simulink model "DUC_filters"  (R2014b)
settings: Solver=FixedStepDiscrete  SolverMode=SingleTasking  StartTime=0.0  StopTime=4096/fs  RelTol=1e-3
PreLoadFcn:
  | %%%%%%%%%%%%%%%%%%%%%%%%%%%%%%%%%%%%%%%%%%%%%%%%%%%%%%%%%%%%%%%%%%%%%%%%%%%
  | % check to see if Simulink library folder is missing from the MATLAB path %
  | %%%%%%%%%%%%%%%%%%%%%%%%%%%%%%%%%%%%%%%%%%%%%%%%%%%%%%%%%%%%%%%%%%%%%%%%%%%
  | if isempty(strfind(path, 'rtlsdr_book_library'))
  | 
  |     % create error window
  |     fig_error = figure(...
  |         'Name', 'Error: RTL-SDR Book Library',...
  |         'Toolbar','none',...
  |         'MenuBar','none',...
  |         'NumberTitle','off',...
  |         'Resize','off',...
  |         'WindowStyle','modal');
  |     fig_error.Position(3) = 600;
  |     fig_error.Position(4) = 150;
  |     fig_axes = axes(...
  |         'Parent',fig_error,...
  |         'Position',[0,0,1,1],...
  |         'visible','off');
  |     % error message
  |     t_title = text(.05,.8,...
  |         'MISSING DIRECTORIES',...
  |         'FontSize',11.5);
  |     t_body = text(.075,.6,...
  |         [{'Simulink cannot find the  \it{<root>}\rm / \it{rtlsdr\_book\_library}\rm  folder in the \it{MATLAB Path}\rm.'},...
  |         {'Please set the MATLAB path following the instructions given in Exercise 2.4.'}],...
  |         'FontSize',10.5);
  |     % buttons
  |     btn_path = uicontrol(...
  |         'Parent',fig_error,...
  |         'String','Set Path Now',...
  |         'FontSize',10,...
  |         'Callback', 'pathtool; close(fig_error);',...
  |         'Position', [fig_error.Position(3)/2-210, 30, 200, 30]);
  |     btn_abort = uicontrol(...
  |         'Parent',fig_error,...
  |         'String','No thanks',...
  |         'FontSize',10,...
  |         'Callback', 'close(fig_error); abort=1;',...
  |         'Position', [fig_error.Position(3)/2+10, 30, 200, 30]);
  | 
  |     % pause to allow user to interact with error box
  |     uiwait(fig_error);
  | 
  |     % abort simulation
  |     try
  |         if abort==1
  |             set_param(gcs, 'SimulationCommand', 'stop');
  |         end
  |     end
  | 
  |     % if user has set path, allow diagram to be updated
  |     if ~exist('abort','var')
  |         % create error window
  |         fig_update = figure(...
  |             'Name', 'Update Diagram',...
  |             'Toolbar','none',...
  |             'MenuBar','none',...
  |             'NumberTitle','off',...
  |             'Resize','off');
  |         fig_update.Position(3) = 400;
  |         fig_update.Position(4) = 120;
  |         fig_axes = axes(...
  |             'Parent',fig_update,...
  |             'Position',[0,0,1,1],...
  |             'visible','off');
  |         % instruction message
  |         t_body = text(.075,.7,...
  |             'Once you have set the path, update the block diagram',...
  |             'FontSize',10.5);
  |         % button
  |         btn_update = uicontrol(...
  |             'Parent',fig_update,...
  |             'String','Update Block Diagram',...
  |             'FontSize',10,...
  |             'Callback', 'set_param(gcs,''SimulationCommand'',''update''); close(gcf)',...
  |             'Position', [fig_update.Position(3)/2-100, 30, 200, 30]);
  |     end
  | 
  |     % clear error components
  |     clear('fig_error','fig_update','fig_axes','t_title','t_body','btn_path','btn_abort','btn_update','abort');
  | 
  | end
  | %%%%%%%%%%%%%%%%%%%%%%%%%%%%%%%%%%%%%%%%%%%%%%%%%%%%%%%%%%%%%%%%%%%%%%%%%%%
  | 
  | DUC1_setup
  | 
  | % annotations for the pink and purple blocks
  | % going from right to left...
  | 
  | MHz = 100;
  | fs = MHz * 1e6;
  | 
  | fs_CIC_in = fs/CIC_R;
  | MHz_CIC_in = MHz/CIC_R;
  | 
  | fs_CFIR_in = fs/(CIC_R*CFIR_L_factor);
  | MHz_CFIR_in = MHz/(CIC_R*CFIR_L_factor);
  | 
  | fs_RRC_in = fs/(CIC_R*CFIR_L_factor*RRC_L_factor);
  | MHz_RRC_in = MHz/(CIC_R*CFIR_L_factor*RRC_L_factor);
StartFcn:
  | close all;
undefined symbols (not defined in the file): CFIR_L_factor, CIC_R, K_cic, RRC_L_factor, startfcn_spectrum_analyzer, startfcn_time_scope
libraries: dspmlti4 x6, rtlsdr_book_library x1, commdigbbndpm3 x1, commrandsrc2 x1, dspsigops x1
CloseFcn:
  | closefcn_model;
Description:
  | Software, Simulation Examples and Design Exercises Licence Agreement
  | 
  | This license agreement refers to the simulation examples, design exercises and files,
  | and associated software MATLAB and Simulink resources that accompany the book:
  | 
  |      Title: Software Defined Radio using MATLAB & Simulink and the RTL-SDR
  |      Published by Strathclyde Academic Media, 2015
  |      Authored by Robert W. Stewart, Kenneth W. Barlee, Dale S.W. Atkinson,
  |      and Louise H. Crockett
  | 
  | and made available as a download from, www.desktopSDR.com or variously acquired
  | by other means such as via USB storage, cloud storage, disk or any other electronic
  | or optical or magnetic storage mechanism. These files and associated software may
  | be used subject to the terms of agreement of the conditions below:
  | 
  |     Copyright © 2015 Robert W. Stewart, Kenneth W. Barlee, Dale S.W. Atkinson,
  |     and Louise H. Crockett
  |     All rights reserved.
  | 
  | Redistribution and use in source and binary forms, with or without modification, are
  | permitted provided that the following conditions are met:
  | 
  |    1.  Redistributions of source code must retain the above copyright notice, this list of
  |         conditions and the following disclaimer.
  | 
  |    2.  Redistributions in binary form must reproduce the above copyright notice, this
  |         list of conditions and the following disclaimer in the documentation and/or other
  |         materials provided with the distribution.
  | 
  |    3.  Neither the name of the copyright holder nor the names of its contributors may
  |         be used to endorse or promote products derived from this software without
  |         specific prior written permission.
  | 
  |    4.  In all cases, the software is, and all modifications and derivatives of the
  |         software shall be, licensed to you solely for use in conjunction with The
  |         MathWorks, Inc. products and service offerings.
  | 
  | THIS SOFTWARE IS PROVIDED BY THE COPYRIGHT HOLDERS AND CONTRIBUTORS
  | "AS IS" AND ANY EXPRESS OR IMPLIED WARRANTIES, INCLUDING, BUT NOT LIMITED
  | TO, THE IMPLIED WARRANTIES OF MERCHANTABILITY AND FITNESS FOR A
  | PARTICULAR PURPOSE ARE DISCLAIMED. IN NO EVENT SHALL THE COPYRIGHT
  | HOLDER OR CONTRIBUTORS BE LIABLE FOR ANY DIRECT, INDIRECT, INCIDENTAL,
  | SPECIAL, EXEMPLARY, OR CONSEQUENTIAL DAMAGES (INCLUDING, BUT NOT
  | LIMITED TO, PROCUREMENT OF SUBSTITUTE GOODS OR SERVICES; LOSS OF USE,
  | DATA, OR PROFITS; OR BUSINESS INTERRUPTION) HOWEVER CAUSED AND ON ANY
  | THEORY OF LIABILITY, WHETHER IN CONTRACT, STRICT LIABILITY, OR TORT
  | (INCLUDING NEGLIGENCE OR OTHERWISE) ARISING IN ANY WAY OUT OF THE USE
  | OF THIS SOFTWARE, EVEN IF ADVISED OF THE POSSIBILITY OF SUCH DAMAGE.
  | 
  | 
  | Audio Tracks used in Simulations Examples and Design Exercises
  | 
  | The music and vocal files used within the Examples files and software within the book
  | were variously written, arranged, performed, recorded and produced by Garrey Rice,
  | Adam Struth, Jamie Struth, Iain Thistlethwaite and also Marshall Craigmyle who
  | collectively, and individually where appropriate, assert and retain all of their copyright,
  | performance and artistic rights. Permission to use and reproduce this music is
  | granted for all purposes associated with MATLAB and Simulink software and the
  | simulation examples and design exercises files that accompany this book. Requests to
  | use the music for any other purpose should be directed to: info@desktopSDR.com.
  | For information on music track names, full credits, and links to the musicians please
  | refer to www.desktopSDR.com/more/audio.
settings Model: Creator=desktopSDR Team  LastModifiedBy=desktopSDR Team
settings DataIOCC: LimitDataPoints=off  SaveOutput=off  SignalLogging=off  SaveTime=off
settings OptimizationCC: BlockReduction=off  ConditionallyExecuteInputs=off  InlineParams=on
settings DebuggingCC: AlgebraicLoopMsg=error  UnderspecifiedInitializationDetection=Classic  MergeDetectMultiDrivingBlocksExec=none  SingleTaskRateTransMsg=error  ParameterOverflowMsg=warning  StateNameClashWarn=warning
settings HardwareCC: ProdHWDeviceType=ASIC/FPGA->ASIC/FPGA  ProdEqTarget=off

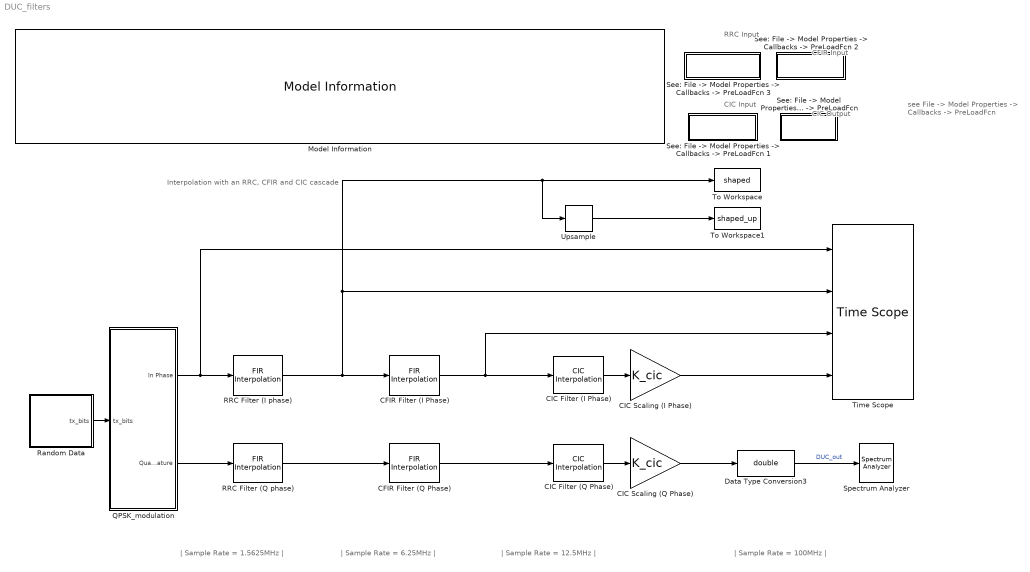
== system DUC_filters ==
  note: | Sample Rate = 1.5625MHz |
  note: Interpolation with an RRC, CFIR and CIC cascade
  note: CIC Input
  note: CIC Output
  note: see File -> Model Properties
      | -> Callbacks -> PreLoadFcn
  note: CFIR Input
  note: RRC Input
  note: | Sample Rate = 6.25MHz |
  note: | Sample Rate = 12.5MHz |
  note: | Sample Rate = 100MHz |
  CFIR Filter (I Phase) : dspmlti4/FIR Interpolation  h=fir1(15,1/4)  L=3  framing=Allow multirate processing  outputBufInitCond=0  firstCoeffDataTypeStr=Inherit: Same word length as input  firstCoeffLastDataTypeStr=Inherit: Same word length as input  firstCoeffMin=[]  firstCoeffMax=[]  outputDataTypeStr=Inherit: Same as accumulator  outputLastDataTypeStr=Inherit: Same as accumulator  outputMin=[]  outputMax=[]  roundingMode=Floor  overflowMode=off  FilterSource=Filter object  FilterObject=hCFIR
  CFIR Filter (Q Phase) : dspmlti4/FIR Interpolation  h=fir1(15,1/4)  L=3  framing=Allow multirate processing  outputBufInitCond=0  firstCoeffDataTypeStr=Inherit: Same word length as input  firstCoeffLastDataTypeStr=Inherit: Same word length as input  firstCoeffMin=[]  firstCoeffMax=[]  outputDataTypeStr=Inherit: Same as accumulator  outputLastDataTypeStr=Inherit: Same as accumulator  outputMin=[]  outputMax=[]  roundingMode=Floor  overflowMode=off  FilterSource=Filter object  FilterObject=hCFIR
  CIC Filter (I Phase) : dspmlti4/CIC Interpolation  filtFrom=Multirate object in workspace  filtobj=hCIC  ftype=Interpolator  R=2  M=1  N=2  filterInternals=Full precision  BPS=[16 16 16 16]  FLPS=0  outputWordLength=32  outputFracLength=0  launchFVT=off  framing=Allow multirate processing
  CIC Filter (Q Phase) : dspmlti4/CIC Interpolation  filtFrom=Multirate object in workspace  filtobj=hCIC  ftype=Interpolator  R=2  M=1  N=2  filterInternals=Full precision  BPS=[16 16 16 16]  FLPS=0  outputWordLength=32  outputFracLength=0  launchFVT=off  framing=Allow multirate processing
  CIC Scaling (I Phase) : Gain  Gain=K_cic  ParamDataTypeStr=fixdt(1,16,15)  OutDataTypeStr=fixdt(1,16,15)
  CIC Scaling (Q Phase) : Gain  Gain=K_cic  ParamDataTypeStr=fixdt(1,16,15)  OutDataTypeStr=fixdt(1,16,15)
  Data Type Conversion3 : DataTypeConversion  OutDataTypeStr=double
  Model Information : rtlsdr_book_library/Additional Tools/Model Information/Model Information
  QPSK_modulation : Subsystem
  RRC Filter (I phase) : dspmlti4/FIR Interpolation  h=fir1(15,1/4)  L=3  framing=Allow multirate processing  outputBufInitCond=0  firstCoeffDataTypeStr=Inherit: Same word length as input  firstCoeffLastDataTypeStr=Inherit: Same word length as input  firstCoeffMin=[]  firstCoeffMax=[]  outputDataTypeStr=Inherit: Same as accumulator  outputLastDataTypeStr=Inherit: Same as accumulator  outputMin=[]  outputMax=[]  roundingMode=Floor  overflowMode=off  FilterSource=Filter object  FilterObject=hRRC
  RRC Filter (Q phase) : dspmlti4/FIR Interpolation  h=fir1(15,1/4)  L=3  framing=Allow multirate processing  outputBufInitCond=0  firstCoeffDataTypeStr=Inherit: Same word length as input  firstCoeffLastDataTypeStr=Inherit: Same word length as input  firstCoeffMin=[]  firstCoeffMax=[]  outputDataTypeStr=Inherit: Same as accumulator  outputLastDataTypeStr=Inherit: Same as accumulator  outputMin=[]  outputMax=[]  roundingMode=Floor  overflowMode=off  FilterSource=Filter object  FilterObject=hRRC
  Random Data : Subsystem
  "See: File -> Model Properties -> Callbacks -> PreLoadFcn " : Subsystem
      mask Display:
      | MHz = evalin('base', 'MHz');
      | fprintf(['fs = ',num2str(MHz),' MHz']);
  "See: File -> Model Properties -> Callbacks -> PreLoadFcn 1" : Subsystem
      mask Display:
      | MHz_CIC_in = evalin('base', 'MHz_CIC_in');
      | fprintf(['fR3 = ',num2str(MHz_CIC_in),' MHz']);
  "See: File -> Model Properties -> Callbacks -> PreLoadFcn 2" : Subsystem
      mask Display:
      | MHz_CFIR_in = evalin('base', 'MHz_CFIR_in');
      | fprintf(['fR2 = ',num2str(MHz_CFIR_in),' MHz']);
  "See: File -> Model Properties -> Callbacks -> PreLoadFcn 3" : Subsystem
      mask Display:
      | MHz_RRC_in = evalin('base', 'MHz_RRC_in');
      | fprintf(['fR1 = ',num2str(MHz_RRC_in),' MHz']);
  Spectrum Analyzer : SpectrumAnalyzer  StartFcn=startfcn_spectrum_analyzer;
  Time Scope : TimeScope  StartFcn=startfcn_time_scope;  DefaultConfigurationName=spbscopes.TimeScopeBlockCfg  NumInputPorts=4
  To Workspace : ToWorkspace  VariableName=shaped  SampleTime=-1
      settings: Save2DSignal=2-D array (concatenate along first dimension)
  To Workspace1 : ToWorkspace  VariableName=shaped_up  SampleTime=-1
      settings: Save2DSignal=2-D array (concatenate along first dimension)
  Upsample : dspsigops/Upsample  N=16  phase=0  InputProcessing=Columns as channels (frame based)  RateOptions=Enforce single-rate processing  ic=0  mode=Unused parameter value
  wires:
  Data Type Conversion3/1 -> Spectrum Analyzer/1  "DUC_out"
  QPSK_modulation/1(In Phase) -> Time Scope/1, RRC Filter (I phase)/1
  RRC Filter (I phase)/1 -> Time Scope/2, Upsample/1, To Workspace/1, CFIR Filter (I Phase)/1
  RRC Filter (Q phase)/1 -> CFIR Filter (Q Phase)/1
  QPSK_modulation/2(Quadrature) -> RRC Filter (Q phase)/1
  CFIR Filter (I Phase)/1 -> CIC Filter (I Phase)/1, Time Scope/3
  CFIR Filter (Q Phase)/1 -> CIC Filter (Q Phase)/1
  CIC Filter (I Phase)/1 -> CIC Scaling (I Phase)/1
  CIC Filter (Q Phase)/1 -> CIC Scaling (Q Phase)/1
  CIC Scaling (I Phase)/1 -> Time Scope/4
  CIC Scaling (Q Phase)/1 -> Data Type Conversion3/1
  Random Data/1(tx_bits) -> QPSK_modulation/1(tx_bits)
  Upsample/1 -> To Workspace1/1

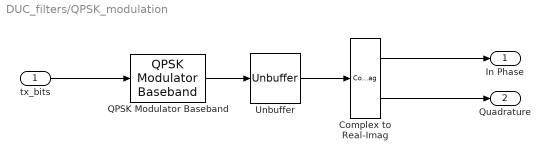
== system DUC_filters/QPSK_modulation ==
  tx_bits : Inport
  Complex to Real-Imag : ComplexToRealImag
  QPSK Modulator Baseband : commdigbbndpm3/QPSK Modulator Baseband  InType=Bit  Enc=Binary  Ph=pi/4  outDtype=Fixed-point  outWordLen=16  outUDDataType=sfix(16)  outFracLenMode=User-defined  outFracLen=15
  Unbuffer : Unbuffer  SampleBasedProcessing=Same as frame based
  In Phase : Outport
  Quadrature : Outport  Port=2
  wires:
  Complex to Real-Imag/2 -> Quadrature/1
  Complex to Real-Imag/1 -> In Phase/1
  QPSK Modulator Baseband/1 -> Unbuffer/1
  tx_bits/1 -> QPSK Modulator Baseband/1
  Unbuffer/1 -> Complex to Real-Imag/1

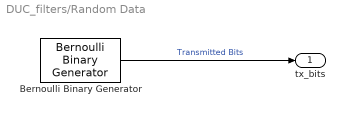
== system DUC_filters/Random Data ==
  Bernoulli Binary Generator : commrandsrc2/Bernoulli Binary Generator  P=0.5  seed=61  Ts=(0.5*CIC_R*RRC_L_factor*CFIR_L_factor)/fs  frameBased=on  sampPerFrame=2  orient=off  outDataType=boolean
  tx_bits : Outport
  wires:
  Bernoulli Binary Generator/1 -> tx_bits/1  "Transmitted Bits"

== system DUC_filters/See: File -> Model Properties -> Callbacks -> PreLoadFcn  ==

== system DUC_filters/See: File -> Model Properties -> Callbacks -> PreLoadFcn 1 ==

== system DUC_filters/See: File -> Model Properties -> Callbacks -> PreLoadFcn 2 ==

== system DUC_filters/See: File -> Model Properties -> Callbacks -> PreLoadFcn 3 ==
